simulink model "mode_select_unit"  (R2023b)
settings: Solver=FixedStepAuto  StartTime=0.0  StopTime=10.0  FixedStep=1e-3  RelTol=1e-3  EnableMultiTasking=on
settings Model: ExtModeTrigDuration=5  Creator=conno  LastModifiedBy=conno
settings OptimizationCC: EnhancedBackFolding=on  PassReuseOutputArgsAs=Individual arguments  ZeroExternalMemoryAtStartup=off  ZeroInternalMemoryAtStartup=off  MaxStackSize=64  OptimizeBlockOrder=speed  DifferentSizesBufferReuse=on  OptimizationCustomize=off  EfficientTunableParamExpr=on
settings DebuggingCC: ParameterTunabilityLossMsg=error
settings HardwareCC: ProdBitPerPointer=32  ProdBitPerSizeT=32  ProdBitPerPtrDiffT=32  ProdLargestAtomicInteger=Long  ProdLargestAtomicFloat=Double  ProdWordSize=32  ProdHWDeviceType=ARM Compatible->ARM Cortex
settings SFSimCC: MATLABDynamicMemAlloc=off
settings RTWCC: Description=Embedded Coder  SystemTargetFile=ert.tlc  HardwareBoard=NXP FRDM-K64F  TLCOptions="-aInlineSetEventsForThisBaseRateFcn=TLC_FALSE -aSuppressMultiTaskScheduler=TLC_FALSE  -aRateBasedStepFcn=0"  TemplateMakefile=ert_default_tmf  Toolchain=GNU Tools for ARM Embedded Processors
settings CodeAppCC: ForceParamTrailComments=on  IgnoreCustomStorageClasses=off  OperatorAnnotations=on  SimulinkDataObjDesc=on  SFDataObjDesc=on  InsertBlockDesc=on
settings ERTTargetCC: ExtModeTransport=4  ExtModeMexFile=sendToCommService

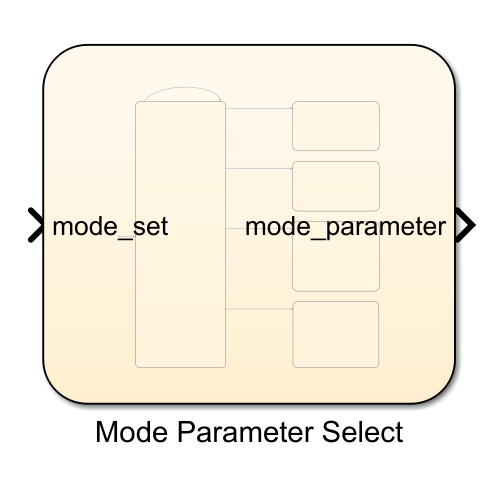
[thumbnail: Simulink's stored preview of the top-level diagram]
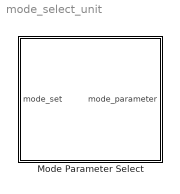
== system mode_select_unit ==
  Mode Parameter Select : Stateflow chart  TreatAsAtomicUnit=on

== stateflow chart mode_select_unit/Mode Parameter Select ==
  state OFF
    % Launch Point for determining mode, takes input
    % and selects proper functionality
    % if no mode selected (MODE 0), wait for it to change
    entry:
    mode_parameter = 0b0000000000000000000000000;
  state AOO
    entry:
    %{
    Parameters Needed:
    LRL
    URL
    Atrial Amplitude
    Atrial Pulse Width
    %}
    mode_parameter = 0b1100001010000000000000000;
  state VOO
    entry:
    %{
    Parameters Needed:
    LRL
    URL
    Ventricular Amplitude
    Ventricular Pulse Width
    %}
    mode_parameter = 0b1100000101000000000000000;
  state AAI
    entry:
    %{
    Parameters Needed:
    Lower Rate Limit
    Upper Rate Limit
    Atrial Amplitude
    Atrial Pulse Width
    Hysteresis
    Rate Smoothing
    Atrial Sensitivity
    ARP
    PVARP
    %}
    mode_parameter = 0b1100001010100110110000000;
  state VVI
    entry:
    %{
    Parameters Needed:
    LRL
    URL
    Ventricle Amplitude
    Ventricle Pulse Width
    Hysteresis
    Rate Smoothing
    Ventricular Sensitivity
    VRP
    %}
    mode_parameter = 0b1100000101011000110000000;
  OFF -> OFF [order 1] : [mode_set == 0]
  OFF -> AOO [order 2] : [mode_set == 1]
  OFF -> VOO [order 3] : [mode_set == 2]
  OFF -> AAI [order 4] : [mode_set == 3]
  (default) -> OFF
  OFF -> VVI [order 5] : [mode_set == 4]
  data: mode_parameter output uint32; mode_set input uint8
